simulink model "controller_arduino"  (R2024a)
settings: Solver=FixedStepDiscrete  StartTime=0.0  StopTime=inf  FixedStep=0.01  RelTol=1e-3  EnableMultiTasking=on
libraries: arduinolib x15, simulink x5
settings Model: ExtModeTrigDuration=2  Creator=DAUIN-Win10  LastModifiedBy=Alizein Khalifeh
settings SolverCC: AutoInsertRateTranBlk=on
settings OptimizationCC: EnhancedBackFolding=on  PassReuseOutputArgsAs=Individual arguments  ZeroExternalMemoryAtStartup=off  ZeroInternalMemoryAtStartup=off  MaxStackSize=64  OptimizeBlockOrder=speed  DifferentSizesBufferReuse=on  OptimizationCustomize=off  EfficientTunableParamExpr=on
settings DebuggingCC: ParameterTunabilityLossMsg=error  UnconnectedInputMsg=warning  UnconnectedOutputMsg=warning  UnconnectedLineMsg=warning
settings HardwareCC: ProdBitPerInt=16  ProdBitPerPointer=16  ProdBitPerSizeT=16  ProdBitPerPtrDiffT=16  ProdLargestAtomicFloat=None  ProdWordSize=8  ProdHWDeviceType=Atmel->AVR
settings ModelReferenceCC: EnableRefExpFcnMdlSchedulingChecks=on
settings SFSimCC: MATLABDynamicMemAlloc=off
settings RTWCC: Description=Embedded Coder  SystemTargetFile=ert.tlc  HardwareBoard=Arduino Uno  PackageGeneratedCodeAndArtifacts=on  TemplateMakefile=ert_default_tmf  Toolchain=Arduino AVR  BuildConfiguration=Faster Runs  GPUComputeCapability=3.5  DLArmComputeVersion=19.05
settings CodeAppCC: ForceParamTrailComments=on  IgnoreCustomStorageClasses=off  OperatorAnnotations=on  SimulinkDataObjDesc=on  SFDataObjDesc=on  InsertBlockDesc=on
settings ERTTargetCC: SupportContinuousTime=on  SupportVariableSizeSignals=on  ExtModeTransport=3  ExtModeStaticAlloc=on  ExtModeStaticAllocSize=250  ExtModeMexFile=ext_xcp  ExtModeIntrfLevel=Level2 - Open

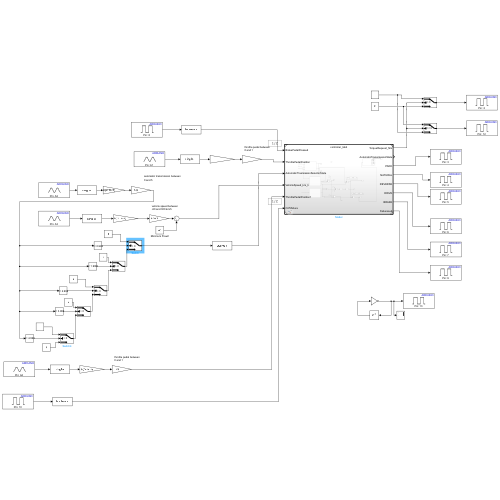
[thumbnail: Simulink's stored preview of the top-level diagram]
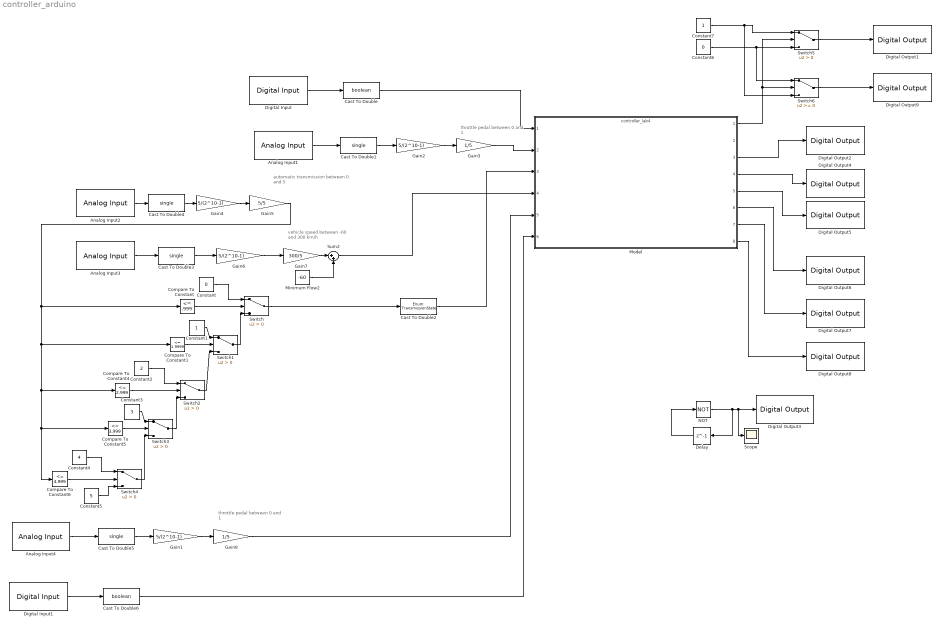
== system controller_arduino ==
  note: throttle pedal between
      | 0 and 1
  note: automatic transmission between
      | 0 and 5
  note: vehicle speed between
      | -60 and 300 km/h
  note: throttle pedal between
      | 0 and 1
  Analog Input1 : arduinolib/Analog Input  pinNumber=1  ReadResultsOnly=off  ConversionTriggerSource=Software  ExternalTriggerType=uint32( 0 )  OutputDataType=uint16  EnableConversionCompleteNotify=off  EnableOuputStatus=off  SampleTime=-1  blockPlatform=arduino
  Analog Input2 : arduinolib/Analog Input  pinNumber=2  ReadResultsOnly=off  ConversionTriggerSource=Software  ExternalTriggerType=uint32( 0 )  OutputDataType=uint16  EnableConversionCompleteNotify=off  EnableOuputStatus=off  SampleTime=-1  blockPlatform=arduino
  Analog Input3 : arduinolib/Analog Input  pinNumber=3  ReadResultsOnly=off  ConversionTriggerSource=Software  ExternalTriggerType=uint32( 0 )  OutputDataType=uint16  EnableConversionCompleteNotify=off  EnableOuputStatus=off  SampleTime=-1  blockPlatform=arduino
  Analog Input4 : arduinolib/Analog Input  pinNumber=4  ReadResultsOnly=off  ConversionTriggerSource=Software  ExternalTriggerType=uint32( 0 )  OutputDataType=uint16  EnableConversionCompleteNotify=off  EnableOuputStatus=off  SampleTime=-1  blockPlatform=arduino
  Cast To Double : DataTypeConversion  OutDataTypeStr=boolean  SaturateOnIntegerOverflow=off  RndMeth=Floor
  Cast To Double{1,3..5} (4 alike) : DataTypeConversion  OutDataTypeStr=single  SaturateOnIntegerOverflow=off  RndMeth=Floor
  Cast To Double2 : DataTypeConversion  OutDataTypeStr=Enum: TransmissionState  SaturateOnIntegerOverflow=off  RndMeth=Floor
  Cast To Double6 : DataTypeConversion  OutDataTypeStr=boolean  SaturateOnIntegerOverflow=off  RndMeth=Floor
  Compare To Constant : simulink/Logic and Bit Operations/Compare To Constant  relop=<=  const=.999  OutDataTypeStr=boolean
  Compare To Constant1 : simulink/Logic and Bit Operations/Compare To Constant  relop=<=  const=1.9999  OutDataTypeStr=boolean
  Compare To Constant4 : simulink/Logic and Bit Operations/Compare To Constant  relop=<=  const=2.999  OutDataTypeStr=boolean
  Compare To Constant5 : simulink/Logic and Bit Operations/Compare To Constant  relop=<=  const=3.999  OutDataTypeStr=boolean
  Compare To Constant6 : simulink/Logic and Bit Operations/Compare To Constant  relop=<=  const=4.999  OutDataTypeStr=boolean
  Constant : Constant  Value=0  OutDataTypeStr=uint16
  Constant1 : Constant  OutDataTypeStr=uint16
  Constant2 : Constant  Value=2  OutDataTypeStr=uint16
  Constant3 : Constant  Value=3  OutDataTypeStr=uint16
  Constant4 : Constant  Value=4  OutDataTypeStr=uint16
  Constant5 : Constant  Value=5  OutDataTypeStr=uint16
  Constant6 : Constant  Value=0  OutDataTypeStr=uint16
  Constant7 : Constant  OutDataTypeStr=uint16
  Delay : Delay  DelayLength=1  SampleTime=0.5
  Digital Input : arduinolib/Digital Input  pinNumber=8  mode=Default  Direction=input  SampleTime=0.1  blockPlatform=arduino
  Digital Input1 : arduinolib/Digital Input  pinNumber=10  mode=Default  Direction=input  SampleTime=0.1  blockPlatform=arduino
  Digital Output1 : arduinolib/Digital Output  pinNumber=2  Direction=output  blockPlatform=arduino
  Digital Output2 : arduinolib/Digital Output  pinNumber=3  Direction=output  blockPlatform=arduino
  Digital Output3 : arduinolib/Digital Output  pinNumber=13  Direction=output  blockPlatform=arduino
  Digital Output4 : arduinolib/Digital Output  pinNumber=4  Direction=output  blockPlatform=arduino
  Digital Output5 : arduinolib/Digital Output  pinNumber=5  Direction=output  blockPlatform=arduino
  Digital Output6 : arduinolib/Digital Output  pinNumber=6  Direction=output  blockPlatform=arduino
  Digital Output7 : arduinolib/Digital Output  pinNumber=7  Direction=output  blockPlatform=arduino
  Digital Output8 : arduinolib/Digital Output  pinNumber=9  Direction=output  blockPlatform=arduino
  Digital Output9 : arduinolib/Digital Output  pinNumber=12  Direction=output  blockPlatform=arduino
  Gain1 : Gain  Gain=5/(2^10-1)
  Gain2 : Gain  Gain=5/(2^10-1)
  Gain3 : Gain  Gain=1/5
  Gain4 : Gain  Gain=5/(2^10-1)  OutDataTypeStr=uint16
  Gain5 : Gain  Gain=5/5  ParamDataTypeStr=uint32  OutDataTypeStr=uint16
  Gain6 : Gain  Gain=5/(2^10-1)
  Gain7 : Gain  Gain=300/5
  Gain8 : Gain  Gain=1/5
  Minimum Flow2 : Constant  Value=-60  OutDataTypeStr=single
  Model : ModelReference  ModelNameDialog=controller_lab4.slx  SimulationMode=Normal  ModelReferenceVersion=6.6
  NOT : Logic  Operator=NOT  IconShape=distinctive  AllPortsSameDT=off  OutDataTypeStr=boolean
  Scope : Scope
  Sum2 : Sum  Inputs=|++
  Switch{,1..5} (6 alike) : Switch  Criteria=u2 > Threshold  SaturateOnIntegerOverflow=off  InputSameDT=off
  Switch6 : Switch  SaturateOnIntegerOverflow=off  InputSameDT=off
  wires:
  Digital Input/1 -> Cast To Double/1
  Cast To Double/1 -> Model/1
  Cast To Double1/1 -> Gain2/1
  Analog Input1/1 -> Cast To Double1/1
  Gain2/1 -> Gain3/1
  NOT/1 -> Delay/1, Scope/1, Digital Output3/1
  Delay/1 -> NOT/1
  Analog Input3/1 -> Cast To Double3/1
  Minimum Flow2/1 -> Sum2/2
  Cast To Double3/1 -> Gain6/1
  Gain6/1 -> Gain7/1
  Gain7/1 -> Sum2/1
  Gain3/1 -> Model/2
  Sum2/1 -> Model/4
  Cast To Double4/1 -> Gain4/1
  Gain4/1 -> Gain5/1
  Compare To Constant/1 -> Switch/2
  Constant/1 -> Switch/1
  Compare To Constant1/1 -> Switch1/2
  Constant1/1 -> Switch1/1
  Switch1/1 -> Switch/3
  Switch3/1 -> Switch2/3
  Compare To Constant5/1 -> Switch3/2
  Constant2/1 -> Switch2/1
  Compare To Constant4/1 -> Switch2/2
  Constant3/1 -> Switch3/1
  Constant4/1 -> Switch4/1
  Compare To Constant6/1 -> Switch4/2
  Switch2/1 -> Switch1/3
  Switch4/1 -> Switch3/3
  Constant5/1 -> Switch4/3
  Cast To Double2/1 -> Model/3
  Switch/1 -> Cast To Double2/1
  Gain5/1 -> Compare To Constant/1, Compare To Constant1/1, Compare To Constant4/1, Compare To Constant5/1, Compare To Constant6/1
  Analog Input2/1 -> Cast To Double4/1
  Gain8/1 -> Model/5
  Cast To Double5/1 -> Gain1/1
  Gain1/1 -> Gain8/1
  Analog Input4/1 -> Cast To Double5/1
  Cast To Double6/1 -> Model/6
  Digital Input1/1 -> Cast To Double6/1
  Model/1 -> Switch6/2, Switch5/2
  Switch5/1 -> Digital Output1/1
  Constant6/1 -> Switch6/1, Switch5/3
  Constant7/1 -> Switch6/3, Switch5/1
  Switch6/1 -> Digital Output9/1
  Model/3 -> Digital Output2/1
  Model/4 -> Digital Output4/1
  Model/5 -> Digital Output5/1
  Model/6 -> Digital Output6/1
  Model/7 -> Digital Output7/1
  Model/8 -> Digital Output8/1
